simulink model "Project1_Part2_Option2_MODEL"  (R2023b)
settings: Solver=VariableStepAuto  StartTime=0.0  StopTime=25  RelTol=1e-3
values from neighbouring files (symbols this model uses):
  A = T_0_values(l)    [Project1_Part2.m]    (also in Project1_Part2_Option1_CODE.m = A_values(j); Project1_Part2_Option2_CODE.m = A_values(j); Project1_Part2_Option3_CODE.m = A_values(j))
  b1 = 1    [Project1_Part2.m]    (also in Project1_Part2_Option1_CODE.m; Project1_Part2_Option2_CODE.m; Project1_Part2_Option3_CODE.m)
  b2 = 1    [Project1_Part2.m]    (also in Project1_Part2_Option1_CODE.m; Project1_Part2_Option2_CODE.m; Project1_Part2_Option3_CODE.m)
  J1 = 100    [Project1_Part2.m]    (also in Project1_Part2_Option1_CODE.m; Project1_Part2_Option2_CODE.m; Project1_Part2_Option3_CODE.m)
  J2 = 1    [Project1_Part2.m]    (also in Project1_Part2_Option1_CODE.m; Project1_Part2_Option2_CODE.m; Project1_Part2_Option3_CODE.m)
settings Model: Creator=turtl  LastModifiedBy=turtl

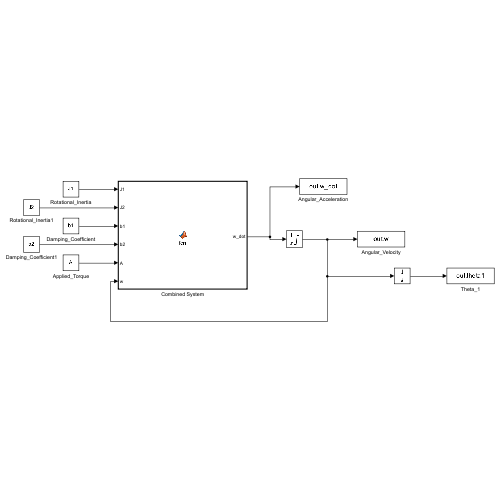
[thumbnail: Simulink's stored preview of the top-level diagram]
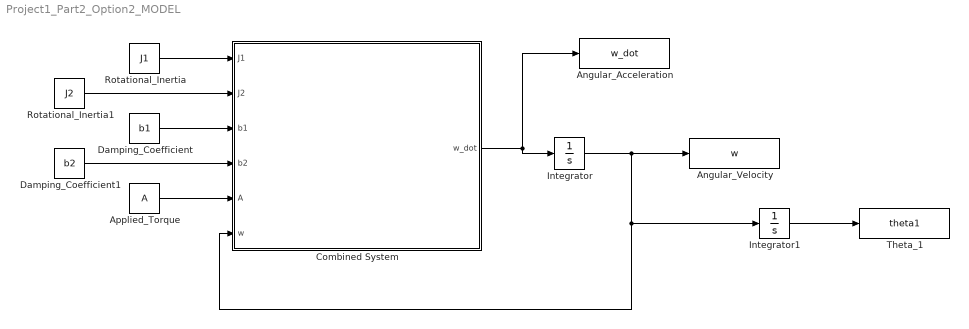
== system Project1_Part2_Option2_MODEL ==
  Angular_Acceleration : ToWorkspace  VariableName=w_dot  SaveFormat=Timeseries  SampleTime=-1
  Angular_Velocity : ToWorkspace  VariableName=w  SaveFormat=Timeseries  SampleTime=-1
  Applied_Torque : Constant  Value=A
  Combined System : MATLAB Function  TreatAsAtomicUnit=on
  Damping_Coefficient : Constant  Value=b1
  Damping_Coefficient1 : Constant  Value=b2
  Integrator : Integrator  LimitOutput=on  UpperSaturationLimit=10000  LowerSaturationLimit=0
  Integrator1 : Integrator
  Rotational_Inertia : Constant  Value=J1
  Rotational_Inertia1 : Constant  Value=J2
  Theta_1 : ToWorkspace  VariableName=theta1  SaveFormat=Timeseries  SampleTime=-1
  wires:
  Applied_Torque/1 -> Combined System/5(A)
  Integrator/1 -> Angular_Velocity/1, Integrator1/1, Combined System/6(w)
  Damping_Coefficient/1 -> Combined System/3(b1)
  Rotational_Inertia/1 -> Combined System/1(J1)
  Integrator1/1 -> Theta_1/1
  Combined System/1(w_dot) -> Angular_Acceleration/1, Integrator/1
  Rotational_Inertia1/1 -> Combined System/2(J2)
  Damping_Coefficient1/1 -> Combined System/4(b2)

== matlab function Project1_Part2_Option2_MODEL/Combined System ==
  data: J1 input; w_dot output; J2 input; b1 input; b2 input; A input; w input
function w_dot = fcn(J1,J2, b1,b2, A,w)
w_dot = (1/(J1+J2))*(A-b1*w-b2*w);
end
